simulink model "Microgrid_GFM_Insular"  (R2025b)
settings: Solver=ode23tb  StartTime=0.0  StopTime=5  MaxStep=1e-5  RelTol=1e-4  AbsTol=1e-6
libraries: spsSeriesRLCBranchLib x8, spsCurrentMeasurementLib x4, spsGroundLib x3, spsVoltageMeasurementLib x3, spsDCVoltageSourceLib x2, spsUniversalBridgeLib x2, spsSeriesRLCLoadLib x2, simulink x2, spsBreakerLib x1, spspowerguiLib x1
settings Model: Creator=Alex  LastModifiedBy=Alex

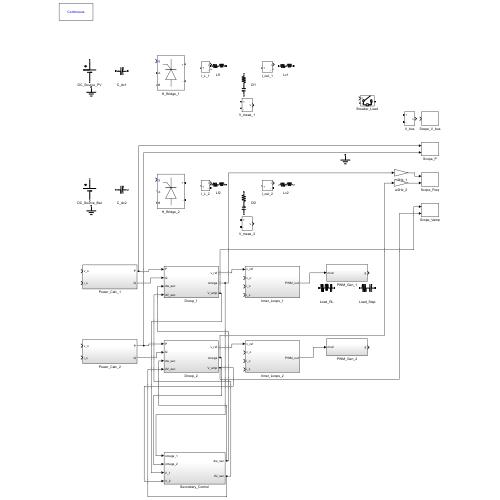
[thumbnail: Simulink's stored preview of the top-level diagram]
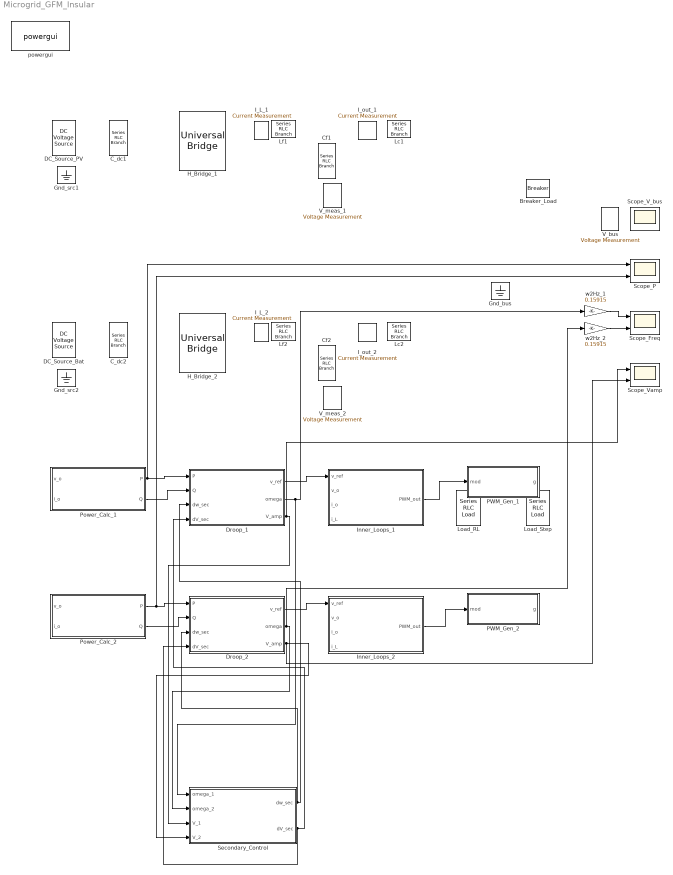
== system Microgrid_GFM_Insular ==
  Breaker_Load : spsBreakerLib/Breaker  InitialState=0  SwitchingTimes=[2]  External=on  BreakerResistance=0.01  SnubberResistance=1e6  SnubberCapacitance=inf  Measurements=None  MoreParameters=on  NoBreakLoop=off
  C_dc1 : spsSeriesRLCBranchLib/Series RLC Branch  LConnTagsString=__new0  RConnTagsString=__new0  BranchType=C  Resistance=1  Inductance=1e-3  SetiL0=off  InitialCurrent=0  Capacitance=1000e-6  Setx0=off  InitialVoltage=0  Measurements=None
  C_dc2 : spsSeriesRLCBranchLib/Series RLC Branch  LConnTagsString=__new0  RConnTagsString=__new0  BranchType=C  Resistance=1  Inductance=1e-3  SetiL0=off  InitialCurrent=0  Capacitance=1000e-6  Setx0=off  InitialVoltage=0  Measurements=None
  Cf1 : spsSeriesRLCBranchLib/Series RLC Branch  LConnTagsString=__new0  RConnTagsString=__new0  BranchType=RC  Resistance=0.01  Inductance=1e-3  SetiL0=off  InitialCurrent=0  Capacitance=2.5e-05  Setx0=off  InitialVoltage=0  Measurements=None
  Cf2 : spsSeriesRLCBranchLib/Series RLC Branch  LConnTagsString=__new0  RConnTagsString=__new0  BranchType=RC  Resistance=0.01  Inductance=1e-3  SetiL0=off  InitialCurrent=0  Capacitance=2.5e-05  Setx0=off  InitialVoltage=0  Measurements=None
  DC_Source_Bat : spsDCVoltageSourceLib/DC Voltage Source  Amplitude=400  Measurements=None
  DC_Source_PV : spsDCVoltageSourceLib/DC Voltage Source  Amplitude=400  Measurements=None
  Droop_1 : Subsystem
  Droop_2 : Subsystem
  Gnd_bus : spsGroundLib/Ground  LConnTagsString=a
  Gnd_src1 : spsGroundLib/Ground  LConnTagsString=a
  Gnd_src2 : spsGroundLib/Ground  LConnTagsString=a
  H_Bridge_1 : spsUniversalBridgeLib/Universal Bridge  Arms=2  SnubberResistance=1e5  SnubberCapacitance=inf  Device=Thyristors  Ron=1e-3  Lon=0  ForwardVoltages="[  0  0  ]"  ForwardVoltage=0  GTOparameters=[ 10e-6 , 20e-6 ]  IGBTparameters=[ 1e-6 , 2e-6 ]  Measurements=None  Measurements_2=None  converterType=Rectifier
  H_Bridge_2 : spsUniversalBridgeLib/Universal Bridge  Arms=2  SnubberResistance=1e5  SnubberCapacitance=inf  Device=Thyristors  Ron=1e-3  Lon=0  ForwardVoltages="[  0  0  ]"  ForwardVoltage=0  GTOparameters=[ 10e-6 , 20e-6 ]  IGBTparameters=[ 1e-6 , 2e-6 ]  Measurements=None  Measurements_2=None  converterType=Rectifier
  I_L_1 : spsCurrentMeasurementLib/Current Measurement  PhasorSimulation=off  OutputType=Complex  PSBequivalent=0
  I_L_2 : spsCurrentMeasurementLib/Current Measurement  PhasorSimulation=off  OutputType=Complex  PSBequivalent=0
  I_out_1 : spsCurrentMeasurementLib/Current Measurement  PhasorSimulation=off  OutputType=Complex  PSBequivalent=0
  I_out_2 : spsCurrentMeasurementLib/Current Measurement  PhasorSimulation=off  OutputType=Complex  PSBequivalent=0
  Inner_Loops_1 : Subsystem
  Inner_Loops_2 : Subsystem
  Lc1 : spsSeriesRLCBranchLib/Series RLC Branch  LConnTagsString=__new0  RConnTagsString=__new0  BranchType=RL  Resistance=0.05  Inductance=0.0005  SetiL0=off  InitialCurrent=0  Capacitance=1e-6  Setx0=off  InitialVoltage=0  Measurements=None
  Lc2 : spsSeriesRLCBranchLib/Series RLC Branch  LConnTagsString=__new0  RConnTagsString=__new0  BranchType=RL  Resistance=0.05  Inductance=0.0005  SetiL0=off  InitialCurrent=0  Capacitance=1e-6  Setx0=off  InitialVoltage=0  Measurements=None
  Lf1 : spsSeriesRLCBranchLib/Series RLC Branch  LConnTagsString=__new0  RConnTagsString=__new0  BranchType=RL  Resistance=0.1  Inductance=0.0025  SetiL0=off  InitialCurrent=0  Capacitance=1e-6  Setx0=off  InitialVoltage=0  Measurements=None
  Lf2 : spsSeriesRLCBranchLib/Series RLC Branch  LConnTagsString=__new0  RConnTagsString=__new0  BranchType=RL  Resistance=0.1  Inductance=0.0025  SetiL0=off  InitialCurrent=0  Capacitance=1e-6  Setx0=off  InitialVoltage=0  Measurements=None
  Load_RL : spsSeriesRLCLoadLib/Series RLC Load  LConnTagsString=a  RConnTagsString=__new0  NominalVoltage=230  NominalFrequency=50  ActivePower=2116  InductivePower=249285.3771  CapacitivePower=100  Setx0=off  InitialVoltage=0  SetiL0=off  InitialCurrent=0  Measurements=None  LoadType=constant Z
  Load_Step : spsSeriesRLCLoadLib/Series RLC Load  LConnTagsString=a  RConnTagsString=__new0  NominalVoltage=230  NominalFrequency=50  ActivePower=1058  InductivePower=0  CapacitivePower=100  Setx0=off  InitialVoltage=0  SetiL0=off  InitialCurrent=0  Measurements=None  LoadType=constant Z
  PWM_Gen_1 : Subsystem
  PWM_Gen_2 : Subsystem
  Power_Calc_1 : Subsystem
  Power_Calc_2 : Subsystem
  Scope_Freq : Scope  NumInputPorts=2
  Scope_P : Scope  NumInputPorts=2
  Scope_V_bus : Scope
  Scope_Vamp : Scope  NumInputPorts=2
  Secondary_Control : Subsystem
  V_bus : spsVoltageMeasurementLib/Voltage Measurement  PhasorSimulation=off  OutputType=Complex  PSBequivalent=0
  V_meas_1 : spsVoltageMeasurementLib/Voltage Measurement  PhasorSimulation=off  OutputType=Complex  PSBequivalent=0
  V_meas_2 : spsVoltageMeasurementLib/Voltage Measurement  PhasorSimulation=off  OutputType=Complex  PSBequivalent=0
  powergui : spspowerguiLib/powergui  Priority=1  SimulationMode=Continuous  SampleTime=50e-6  frequency=60  Iterations=50  frequencyindice=60  Pbase=100e6  ErrMax=1e-4  UnitsV=kV  UnitsW=MW  buscounter=0  FunctionMessages=off  echomessages=off  EnableUseOfTLC=off  CurrentSourceSwitches=off  DisableSnubberDevices=off  DisableRonSwitches=off  DisableVfSwitches=off  DisplayEquations=off  AutomaticDiscreteSolvers=off  SolverType=Tustin/Backward Euler (TBE)  Interpol=off  ExternalGateDelay=off  methode=off  Ts=100  x0status=blocks  SPID=on  SwTol=0  HookPort=off  NonlinearTolerance=1e-4  nMaxIteration=100  ContinueOnMaxIteration=off  RestoreLinks=warning  ResistiveCurrentMeasurement=off  Frange=[0:2:500]  Ylog=off  Xlog=on  ShowGrid=off  save=off  variable=ZData  structure=0  ZoomFFT=off  StartTime=0.0  cycles=1  DisplayStyle=1  fundamental=60  FreqAxis=off  MaxFrequency=1000  frequencyindicesteady=1  RmsSteady=1  display=off
  w2Hz_1 : Gain  Gain=0.15915
  w2Hz_2 : Gain  Gain=0.15915
  wires:
  Power_Calc_1/1(P) -> Droop_1/1(P), Scope_P/1
  Power_Calc_1/2(Q) -> Droop_1/2(Q)
  Droop_1/1(v_ref) -> Inner_Loops_1/1(v_ref)
  Inner_Loops_1/1(PWM_out) -> PWM_Gen_1/1(mod)
  Power_Calc_2/1(P) -> Droop_2/1(P), Scope_P/2
  Power_Calc_2/2(Q) -> Droop_2/2(Q)
  Droop_2/1(v_ref) -> Inner_Loops_2/1(v_ref)
  Inner_Loops_2/1(PWM_out) -> PWM_Gen_2/1(mod)
  Droop_1/2(omega) -> Secondary_Control/1(omega_1), w2Hz_1/1
  Droop_2/2(omega) -> Secondary_Control/2(omega_2), w2Hz_2/1
  Droop_1/3(V_amp) -> Secondary_Control/3(V_1), Scope_Vamp/1
  Droop_2/3(V_amp) -> Secondary_Control/4(V_2), Scope_Vamp/2
  Secondary_Control/1(dw_sec) -> Droop_1/3(dw_sec), Droop_2/3(dw_sec)
  Secondary_Control/2(dV_sec) -> Droop_1/4(dV_sec), Droop_2/4(dV_sec)
  w2Hz_1/1 -> Scope_Freq/1
  w2Hz_2/1 -> Scope_Freq/2

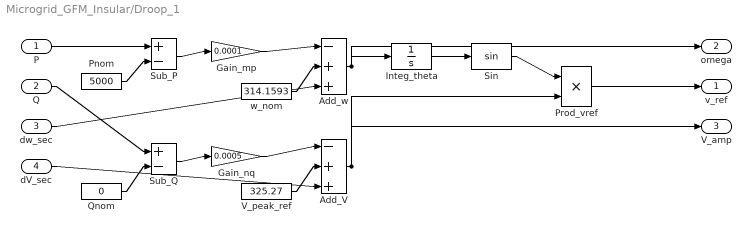
== system Microgrid_GFM_Insular/Droop_1 ==
  P : Inport
  Q : Inport  Port=2
  dw_sec : Inport  Port=3
  dV_sec : Inport  Port=4
  Add_V : Sum  Inputs=-++
  Add_w : Sum  Inputs=-++
  Gain_mp : Gain  Gain=0.0001
  Gain_nq : Gain  Gain=0.0005
  Integ_theta : Integrator
  Pnom : Constant  Value=5000
  Prod_vref : Product
  Qnom : Constant  Value=0
  Sin : Trigonometry
  Sub_P : Sum  Inputs=+-
  Sub_Q : Sum  Inputs=+-
  V_peak_ref : Constant  Value=325.27
  w_nom : Constant  Value=314.1593
  v_ref : Outport
  omega : Outport  Port=2
  V_amp : Outport  Port=3
  wires:
  P/1 -> Sub_P/1
  Pnom/1 -> Sub_P/2
  Sub_P/1 -> Gain_mp/1
  Gain_mp/1 -> Add_w/1
  w_nom/1 -> Add_w/2
  dw_sec/1 -> Add_w/3
  Q/1 -> Sub_Q/1
  Qnom/1 -> Sub_Q/2
  Sub_Q/1 -> Gain_nq/1
  Gain_nq/1 -> Add_V/1
  V_peak_ref/1 -> Add_V/2
  dV_sec/1 -> Add_V/3
  Add_w/1 -> Integ_theta/1, omega/1
  Integ_theta/1 -> Sin/1
  Sin/1 -> Prod_vref/1
  Add_V/1 -> Prod_vref/2, V_amp/1
  Prod_vref/1 -> v_ref/1

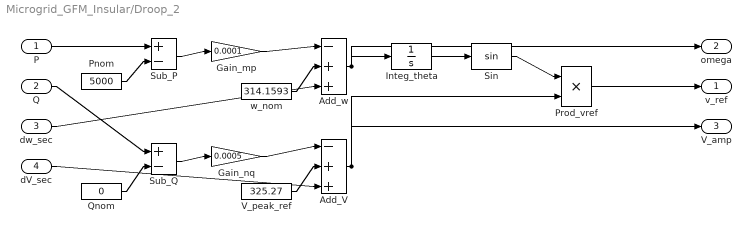
== system Microgrid_GFM_Insular/Droop_2 ==
  P : Inport
  Q : Inport  Port=2
  dw_sec : Inport  Port=3
  dV_sec : Inport  Port=4
  Add_V : Sum  Inputs=-++
  Add_w : Sum  Inputs=-++
  Gain_mp : Gain  Gain=0.0001
  Gain_nq : Gain  Gain=0.0005
  Integ_theta : Integrator
  Pnom : Constant  Value=5000
  Prod_vref : Product
  Qnom : Constant  Value=0
  Sin : Trigonometry
  Sub_P : Sum  Inputs=+-
  Sub_Q : Sum  Inputs=+-
  V_peak_ref : Constant  Value=325.27
  w_nom : Constant  Value=314.1593
  v_ref : Outport
  omega : Outport  Port=2
  V_amp : Outport  Port=3
  wires:
  P/1 -> Sub_P/1
  Pnom/1 -> Sub_P/2
  Sub_P/1 -> Gain_mp/1
  Gain_mp/1 -> Add_w/1
  w_nom/1 -> Add_w/2
  dw_sec/1 -> Add_w/3
  Q/1 -> Sub_Q/1
  Qnom/1 -> Sub_Q/2
  Sub_Q/1 -> Gain_nq/1
  Gain_nq/1 -> Add_V/1
  V_peak_ref/1 -> Add_V/2
  dV_sec/1 -> Add_V/3
  Add_w/1 -> Integ_theta/1, omega/1
  Integ_theta/1 -> Sin/1
  Sin/1 -> Prod_vref/1
  Add_V/1 -> Prod_vref/2, V_amp/1
  Prod_vref/1 -> v_ref/1

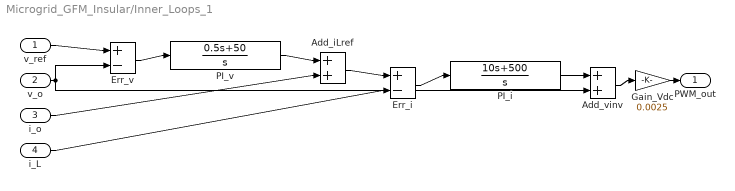
== system Microgrid_GFM_Insular/Inner_Loops_1 ==
  v_ref : Inport
  v_o : Inport  Port=2
  i_o : Inport  Port=3
  i_L : Inport  Port=4
  Add_iLref : Sum
  Add_vinv : Sum
  Err_i : Sum  Inputs=+-
  Err_v : Sum  Inputs=+-
  Gain_Vdc : Gain  Gain=0.0025
  PI_i : TransferFcn  Numerator=[10 500]  Denominator=[1 0]
  PI_v : TransferFcn  Numerator=[0.5 50]  Denominator=[1 0]
  PWM_out : Outport
  wires:
  v_ref/1 -> Err_v/1
  v_o/1 -> Err_v/2, Add_vinv/2
  Err_v/1 -> PI_v/1
  PI_v/1 -> Add_iLref/1
  i_o/1 -> Add_iLref/2
  Add_iLref/1 -> Err_i/1
  i_L/1 -> Err_i/2
  Err_i/1 -> PI_i/1
  PI_i/1 -> Add_vinv/1
  Add_vinv/1 -> Gain_Vdc/1
  Gain_Vdc/1 -> PWM_out/1

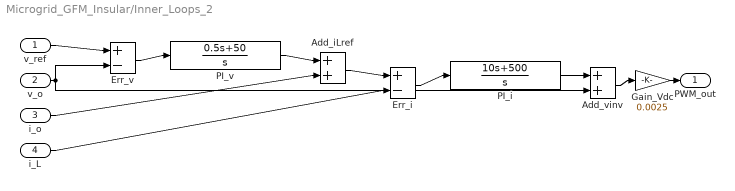
== system Microgrid_GFM_Insular/Inner_Loops_2 ==
  v_ref : Inport
  v_o : Inport  Port=2
  i_o : Inport  Port=3
  i_L : Inport  Port=4
  Add_iLref : Sum
  Add_vinv : Sum
  Err_i : Sum  Inputs=+-
  Err_v : Sum  Inputs=+-
  Gain_Vdc : Gain  Gain=0.0025
  PI_i : TransferFcn  Numerator=[10 500]  Denominator=[1 0]
  PI_v : TransferFcn  Numerator=[0.5 50]  Denominator=[1 0]
  PWM_out : Outport
  wires:
  v_ref/1 -> Err_v/1
  v_o/1 -> Err_v/2, Add_vinv/2
  Err_v/1 -> PI_v/1
  PI_v/1 -> Add_iLref/1
  i_o/1 -> Add_iLref/2
  Add_iLref/1 -> Err_i/1
  i_L/1 -> Err_i/2
  Err_i/1 -> PI_i/1
  PI_i/1 -> Add_vinv/1
  Add_vinv/1 -> Gain_Vdc/1
  Gain_Vdc/1 -> PWM_out/1

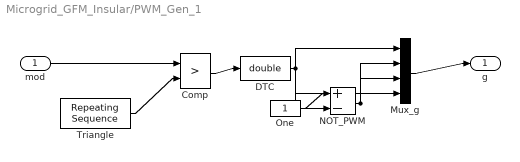
== system Microgrid_GFM_Insular/PWM_Gen_1 ==
  mod : Inport
  Comp : RelationalOperator  Operator=>  OutDataTypeStr=boolean  RndMeth=Simplest  InputSameDT=off
  DTC : DataTypeConversion  OutDataTypeStr=double  SaturateOnIntegerOverflow=off  RndMeth=Floor
  Mux_g : Mux
  NOT_PWM : Sum  Inputs=+-
  One : Constant
  Triangle : simulink/Sources/Repeating Sequence  rep_seq_t=[0 5e-05 0.0001]  rep_seq_y=[-1 1 -1]
  g : Outport
  wires:
  mod/1 -> Comp/1
  Triangle/1 -> Comp/2
  Comp/1 -> DTC/1
  One/1 -> NOT_PWM/1
  DTC/1 -> NOT_PWM/2, Mux_g/1, Mux_g/4
  NOT_PWM/1 -> Mux_g/2, Mux_g/3
  Mux_g/1 -> g/1

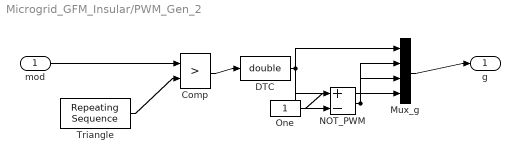
== system Microgrid_GFM_Insular/PWM_Gen_2 ==
  mod : Inport
  Comp : RelationalOperator  Operator=>  OutDataTypeStr=boolean  RndMeth=Simplest  InputSameDT=off
  DTC : DataTypeConversion  OutDataTypeStr=double  SaturateOnIntegerOverflow=off  RndMeth=Floor
  Mux_g : Mux
  NOT_PWM : Sum  Inputs=+-
  One : Constant
  Triangle : simulink/Sources/Repeating Sequence  rep_seq_t=[0 5e-05 0.0001]  rep_seq_y=[-1 1 -1]
  g : Outport
  wires:
  mod/1 -> Comp/1
  Triangle/1 -> Comp/2
  Comp/1 -> DTC/1
  One/1 -> NOT_PWM/1
  DTC/1 -> NOT_PWM/2, Mux_g/1, Mux_g/4
  NOT_PWM/1 -> Mux_g/2, Mux_g/3
  Mux_g/1 -> g/1

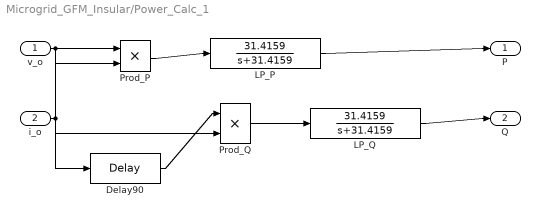
== system Microgrid_GFM_Insular/Power_Calc_1 ==
  v_o : Inport
  i_o : Inport  Port=2
  Delay90 : TransportDelay  DelayTime=0.005
  LP_P : TransferFcn  Numerator=[31.4159]  Denominator=[1 31.4159]
  LP_Q : TransferFcn  Numerator=[31.4159]  Denominator=[1 31.4159]
  Prod_P : Product
  Prod_Q : Product
  P : Outport
  Q : Outport  Port=2
  wires:
  v_o/1 -> Prod_P/1, Delay90/1
  i_o/1 -> Prod_P/2, Prod_Q/2
  Prod_P/1 -> LP_P/1
  LP_P/1 -> P/1
  Delay90/1 -> Prod_Q/1
  Prod_Q/1 -> LP_Q/1
  LP_Q/1 -> Q/1

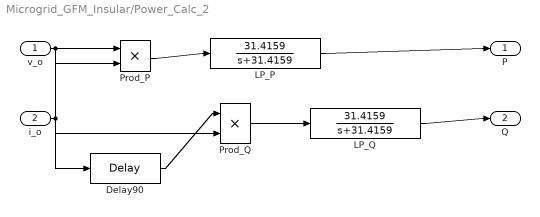
== system Microgrid_GFM_Insular/Power_Calc_2 ==
  v_o : Inport
  i_o : Inport  Port=2
  Delay90 : TransportDelay  DelayTime=0.005
  LP_P : TransferFcn  Numerator=[31.4159]  Denominator=[1 31.4159]
  LP_Q : TransferFcn  Numerator=[31.4159]  Denominator=[1 31.4159]
  Prod_P : Product
  Prod_Q : Product
  P : Outport
  Q : Outport  Port=2
  wires:
  v_o/1 -> Prod_P/1, Delay90/1
  i_o/1 -> Prod_P/2, Prod_Q/2
  Prod_P/1 -> LP_P/1
  LP_P/1 -> P/1
  Delay90/1 -> Prod_Q/1
  Prod_Q/1 -> LP_Q/1
  LP_Q/1 -> Q/1

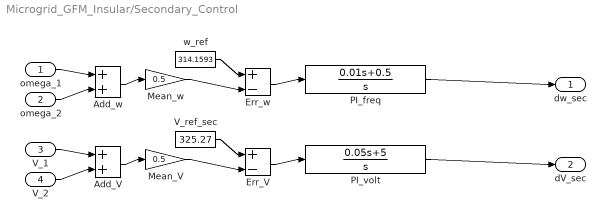
== system Microgrid_GFM_Insular/Secondary_Control ==
  omega_1 : Inport
  omega_2 : Inport  Port=2
  V_1 : Inport  Port=3
  V_2 : Inport  Port=4
  Add_V : Sum
  Add_w : Sum
  Err_V : Sum  Inputs=+-
  Err_w : Sum  Inputs=+-
  Mean_V : Gain  Gain=0.5
  Mean_w : Gain  Gain=0.5
  PI_freq : TransferFcn  Numerator=[0.01 0.5]  Denominator=[1 0]
  PI_volt : TransferFcn  Numerator=[0.05 5]  Denominator=[1 0]
  V_ref_sec : Constant  Value=325.27
  w_ref : Constant  Value=314.1593
  dw_sec : Outport
  dV_sec : Outport  Port=2
  wires:
  omega_1/1 -> Add_w/1
  omega_2/1 -> Add_w/2
  Add_w/1 -> Mean_w/1
  w_ref/1 -> Err_w/1
  Mean_w/1 -> Err_w/2
  Err_w/1 -> PI_freq/1
  PI_freq/1 -> dw_sec/1
  V_1/1 -> Add_V/1
  V_2/1 -> Add_V/2
  Add_V/1 -> Mean_V/1
  V_ref_sec/1 -> Err_V/1
  Mean_V/1 -> Err_V/2
  Err_V/1 -> PI_volt/1
  PI_volt/1 -> dV_sec/1
